simulink model "X_MEGA2560_ADVOneWire_task"  (Simulink 7.0)
libraries: logiclib x81, mathlib x64, analoglib x12, genlib x4, arclib x2, speclib x1
settings Model: Creator=Jarda  LastModifiedBy=Jarda  ExtModeTrigMode=oneshot  ExtModeArmWhenConnect=off

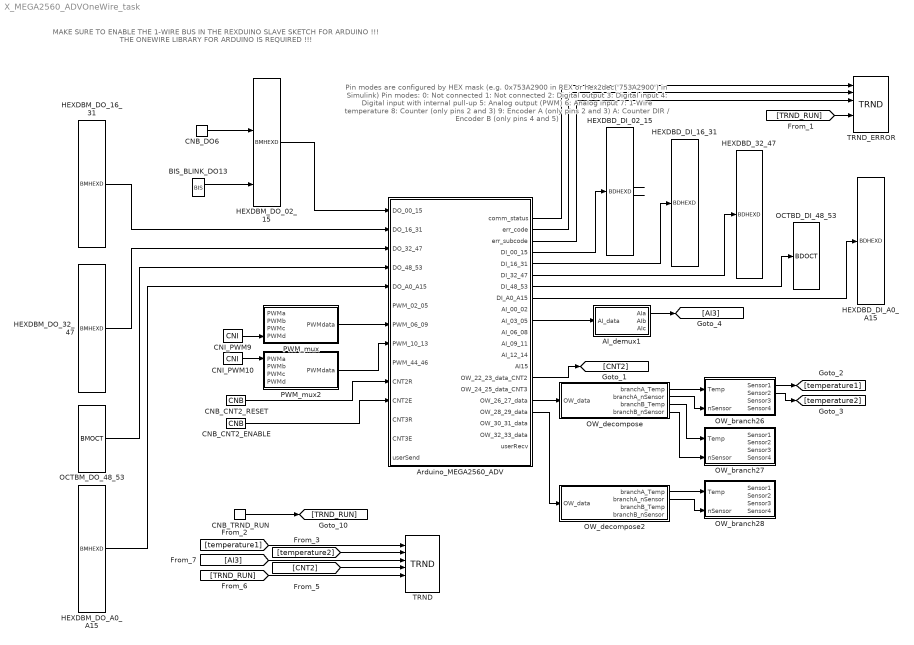
== system X_MEGA2560_ADVOneWire_task ==
  note: Pin modes are configured by HEX mask
      |    (e.g. 0x753A2900 in REX or hex2dec('753A2900') in Simulink)
      |
      | Pin modes:
      | 0: Not connected
      | 1: Not connected
      | 2: Digital output
      | 3: Digital input
      | 4: Digital input with internal pull-up
      | 5: Analog output (PWM)
      | 6: Analog input
      | 7: 1-Wire temperature
      | 8: Counter (only pins 2 and 3)
      | 9: Encoder A (only pins 2 and 3)
      | A: Counter DIR / Encoder B (only pins 4 and 5)
  note: MAKE SURE TO ENABLE THE 1-WIRE BUS IN
      | THE REXDUINO SLAVE SKETCH FOR ARDUINO !!!
      |
      | THE ONEWIRE LIBRARY FOR ARDUINO IS REQUIRED !!!
  AI_demux1 : Subsystem
      mask Type: REX sequence
  Arduino_MEGA2560_ADV : Subsystem  mask(REX sequence){comPort=/dev/ttyACM0, pinmodes_00_07=0x320A0800, pinmodes_08_15=0x00200554, pinmodes_16_23=0, pinmodes_24_31=0x00077700, pinmodes_32_39=0, pinmodes_40_47=0, pinmodes_48_53=0, pinmodes_A0_A7=0x00006000, pinmodes_A8_A15=0}
      mask prompts: comPort "Serial device, e.g. COM7, /dev/ttyACM0, /dev/ttyUSB0 etc."; pinmodes_00_07 "Pin modes 0 to 7 (0 and 1 ignored)"; pinmodes_08_15 "Pin modes 8 to 15"; pinmodes_16_23 "Pin modes 16 to 23"; pinmodes_24_31 "Pin modes 24 to 31"; pinmodes_32_39 "Pin modes 32 to 39"; pinmodes_40_47 "Pin modes 40 to 47"; pinmodes_48_53 "Pin modes 48 to 53"; pinmodes_A0_A7 "Pin modes A0 to A7"; pinmodes_A8_A15 "Pin modes A8 to A15"
      mask CallbackString:
      | REXduino_mask_comPort = get_param(gcb,'comPort');
      | REXduino_mask_comPort = sscanf(fliplr(REXduino_mask_comPort),'%u',1);
      | if ( ~isempty(REXduino_mask_comPort) & (REXduino_mask_comPort<100) )
      | set_param([gcb '/CNI_comPort'],'icn',fliplr(num2str(REXduino_mask_comPort)))
      | else
      | set_param([gcb '/CNI_comPort'],'icn','15')
      | end
      | clear REXduino_mask_comPort|||||||||
  BIS_BLINK_DO13 : genlib/BIS  Y0=off  t1=2  t2=4  t3=0  t4=4  t5=5  t6=6  t7=7  t8=8  RPT=on
  CNB_CNT2_ENABLE : mathlib/CNB  YCN=on
  CNB_CNT2_RESET : mathlib/CNB  YCN=off
  CNB_DO6 : mathlib/CNB  YCN=on
  CNB_TRND_RUN : mathlib/CNB  YCN=on
  CNI_PWM10 : mathlib/CNI  icn=128
  CNI_PWM9 : mathlib/CNI  icn=128
  HEXDBD_32_47 : logiclib/BDHEXD  shift=0
  HEXDBD_DI_02_15 : logiclib/BDHEXD  shift=0
  HEXDBD_DI_16_31 : logiclib/BDHEXD  shift=0
  HEXDBD_DI_A0_A15 : logiclib/BDHEXD  shift=0
  HEXDBM_DO_02_15 : logiclib/BMHEXD  shift=0
  HEXDBM_DO_16_31 : logiclib/BMHEXD  shift=0
  HEXDBM_DO_32_47 : logiclib/BMHEXD  shift=0
  HEXDBM_DO_A0_A15 : logiclib/BMHEXD  shift=0
  OCTBD_DI_48_53 : logiclib/BDOCT  shift=0
  OCTBM_DO_48_53 : logiclib/BMOCT  shift=0
  OW_branch26 : Subsystem
      mask Type: REX sequence
  OW_branch27 : Subsystem
      mask Type: REX sequence
  OW_branch28 : Subsystem
      mask Type: REX sequence
  OW_decompose : Subsystem
      mask Type: REX sequence
  OW_decompose2 : Subsystem
      mask Type: REX sequence
  PWM_mux : Subsystem
      mask Type: REX sequence
  PWM_mux2 : Subsystem
      mask Type: REX sequence
  TRND : arclib/TRND  n=4  l=14400  btype=8: Double  ptype1=1: Store  ptype2=1: Store  ptype3=1: Store  ptype4=1: Store  pfac=1  afac=0  arc=0  id=1  Title=Data trend
  TRND_ERROR : arclib/TRND  n=4  l=1000  btype=8: Double  ptype1=1: Store  ptype2=1: Store  ptype3=1: Store  ptype4=1: Store  pfac=1  afac=0  arc=0  id=1  Title=ERROR trend
  wires:
  AI_demux1/1(AIa) -> [AI3]
  Arduino_MEGA2560_ADV/1(comm_status) -> TRND_ERROR/1
  Arduino_MEGA2560_ADV/2(err_code) -> TRND_ERROR/2
  Arduino_MEGA2560_ADV/3(err_subcode) -> TRND_ERROR/3
  Arduino_MEGA2560_ADV/4(DI_00_15) -> HEXDBD_DI_02_15/1
  Arduino_MEGA2560_ADV/5(DI_16_31) -> HEXDBD_DI_16_31/1
  Arduino_MEGA2560_ADV/6(DI_32_47) -> HEXDBD_32_47/1
  Arduino_MEGA2560_ADV/7(DI_48_53) -> OCTBD_DI_48_53/1
  Arduino_MEGA2560_ADV/8(DI_A0_A15) -> HEXDBD_DI_A0_A15/1
  Arduino_MEGA2560_ADV/10(AI_03_05) -> AI_demux1/1(AI_data)
  Arduino_MEGA2560_ADV/15(OW_22_23_data_CNT2) -> [CNT2]
  Arduino_MEGA2560_ADV/17(OW_26_27_data) -> OW_decompose/1(OW_data)
  Arduino_MEGA2560_ADV/18(OW_28_29_data) -> OW_decompose2/1(OW_data)
  BIS_BLINK_DO13/1 -> HEXDBM_DO_02_15/14
  CNB_CNT2_ENABLE/1 -> Arduino_MEGA2560_ADV/11(CNT2E)
  CNB_CNT2_RESET/1 -> Arduino_MEGA2560_ADV/10(CNT2R)
  CNB_DO6/1 -> HEXDBM_DO_02_15/7
  CNB_TRND_RUN/1 -> [TRND_RUN]
  CNI_PWM10/1 -> PWM_mux2/1(PWMa)
  CNI_PWM9/1 -> PWM_mux/4(PWMd)
  [TRND_RUN] -> TRND_ERROR/5
  [temperature1] -> TRND/1
  [temperature2] -> TRND/2
  [CNT2] -> TRND/4
  [TRND_RUN] -> TRND/5
  [AI3] -> TRND/3
  HEXDBD_DI_02_15/8 -> ?
  HEXDBD_DI_02_15/9 -> ?
  HEXDBM_DO_02_15/1 -> Arduino_MEGA2560_ADV/1(DO_00_15)
  HEXDBM_DO_16_31/1 -> Arduino_MEGA2560_ADV/2(DO_16_31)
  HEXDBM_DO_32_47/1 -> Arduino_MEGA2560_ADV/3(DO_32_47)
  HEXDBM_DO_A0_A15/1 -> Arduino_MEGA2560_ADV/5(DO_A0_A15)
  OCTBM_DO_48_53/1 -> Arduino_MEGA2560_ADV/4(DO_48_53)
  OW_branch26/1(Sensor1) -> [temperature1]
  OW_branch26/2(Sensor2) -> [temperature2]
  OW_decompose/1(branchA_Temp) -> OW_branch26/1(Temp)
  OW_decompose/2(branchA_nSensor) -> OW_branch26/2(nSensor)
  OW_decompose/3(branchB_Temp) -> OW_branch27/1(Temp)
  OW_decompose/4(branchB_nSensor) -> OW_branch27/2(nSensor)
  OW_decompose2/1(branchA_Temp) -> OW_branch28/1(Temp)
  OW_decompose2/2(branchA_nSensor) -> OW_branch28/2(nSensor)
  PWM_mux/1(PWMdata) -> Arduino_MEGA2560_ADV/7(PWM_06_09)
  PWM_mux2/1(PWMdata) -> Arduino_MEGA2560_ADV/8(PWM_10_13)

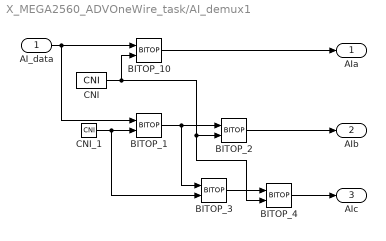
== system X_MEGA2560_ADVOneWire_task/AI_demux1 ==
  AI_data : Inport  Port=1
  BITOP_1 : logiclib/BITOP  iop=6: Shift Right
  BITOP_10 : logiclib/BITOP  iop=3: Bit AND
  BITOP_2 : logiclib/BITOP  iop=3: Bit AND
  BITOP_3 : logiclib/BITOP  iop=6: Shift Right
  BITOP_4 : logiclib/BITOP  iop=3: Bit AND
  CNI : mathlib/CNI  icn=1023
  CNI_1 : mathlib/CNI  icn=10
  AIa : Outport  Port=1
  AIb : Outport  Port=2
  AIc : Outport  Port=3
  wires:
  AI_data/1 -> BITOP_1/1, BITOP_10/1
  BITOP_1/1 -> BITOP_2/1, BITOP_3/1
  BITOP_10/1 -> AIa/1
  BITOP_2/1 -> AIb/1
  BITOP_3/1 -> BITOP_4/1
  BITOP_4/1 -> AIc/1
  CNI/1 -> BITOP_10/2, BITOP_2/2, BITOP_4/2
  CNI_1/1 -> BITOP_1/2, BITOP_3/2

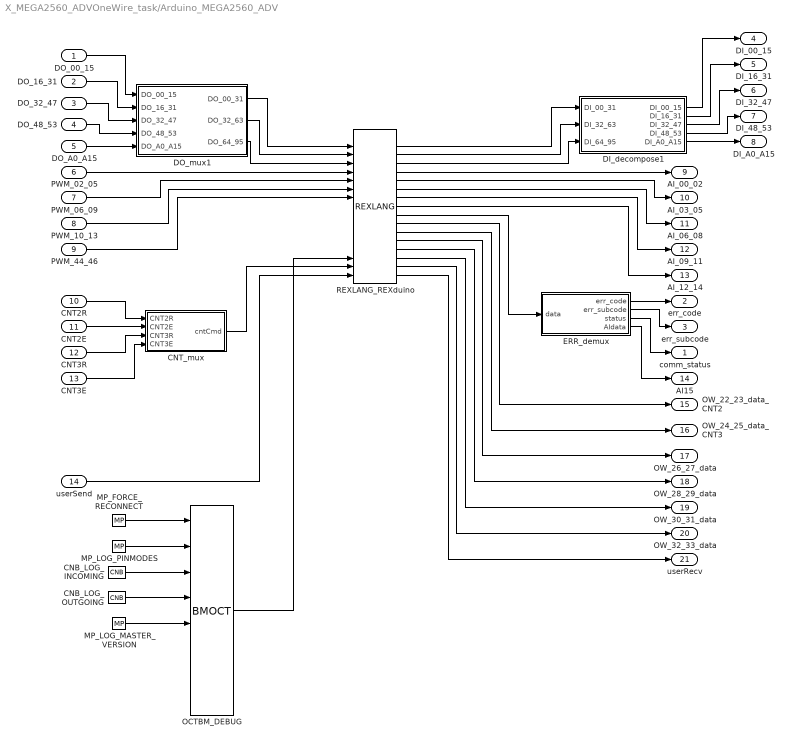
== system X_MEGA2560_ADVOneWire_task/Arduino_MEGA2560_ADV ==
  DO_00_15 : Inport  Port=1  PortWidth=-1  SampleTime=-1  DataType=auto
      settings: SignalType=auto
  DO_16_31 : Inport  Port=2  PortWidth=-1  SampleTime=-1  DataType=auto
      settings: SignalType=auto
  DO_32_47 : Inport  Port=3  PortWidth=-1  SampleTime=-1  DataType=auto
      settings: SignalType=auto
  DO_48_53 : Inport  Port=4  PortWidth=-1  SampleTime=-1  DataType=auto
      settings: SignalType=auto
  DO_A0_A15 : Inport  Port=5  PortWidth=-1  SampleTime=-1  DataType=auto
      settings: SignalType=auto
  PWM_02_05 : Inport  Port=6  PortWidth=-1  SampleTime=-1  DataType=auto
      settings: SignalType=auto
  PWM_06_09 : Inport  Port=7  PortWidth=-1  SampleTime=-1  DataType=auto
      settings: SignalType=auto
  PWM_10_13 : Inport  Port=8  PortWidth=-1  SampleTime=-1  DataType=auto
      settings: SignalType=auto
  PWM_44_46 : Inport  Port=9  PortWidth=-1  SampleTime=-1  DataType=auto
      settings: SignalType=auto
  CNT2R : Inport  Port=10  PortWidth=-1  SampleTime=-1  DataType=auto
      settings: SignalType=auto
  CNT2E : Inport  Port=11  PortWidth=-1  SampleTime=-1  DataType=auto
      settings: SignalType=auto
  CNT3R : Inport  Port=12  PortWidth=-1  SampleTime=-1  DataType=auto
      settings: SignalType=auto
  CNT3E : Inport  Port=13  PortWidth=-1  SampleTime=-1  DataType=auto
      settings: SignalType=auto
  userSend : Inport  Port=14  PortWidth=-1  SampleTime=-1  DataType=auto
      settings: SignalType=auto
  CNB_LOG_INCOMING : mathlib/CNB  SystemSampleTime=-1  YCN=off
  CNB_LOG_OUTGOING : mathlib/CNB  SystemSampleTime=-1  YCN=off
  CNT_mux : Subsystem
      mask Type: REX sequence
  DI_decompose1 : Subsystem
      mask Type: REX sequence
  DO_mux1 : Subsystem
      mask Type: REX sequence
  ERR_demux : Subsystem
      mask Type: REX sequence
  MP_FORCE_RECONNECT : genlib/MP  SystemSampleTime=-1  pwidth=10  BSTATE=off  RPTF=off
  MP_LOG_MASTER_VERSION : genlib/MP  SystemSampleTime=-1  pwidth=10  BSTATE=off  RPTF=off
  MP_LOG_PINMODES : genlib/MP  SystemSampleTime=-1  pwidth=10  BSTATE=off  RPTF=off
  OCTBM_DEBUG : logiclib/BMOCT  SystemSampleTime=-1  shift=0
  REXLANG_REXduino : speclib/REXLANG  tab_matlab=MORE  srcname=REXduino_master.stl  srctype=1: STL  stack=0  debug=1: No check  fname=comPort  p0=0  p1=pinmodes_00_07  p2=pinmodes_08_15  p3=pinmodes_16_23  p4=pinmodes_24_31  p5=pinmodes_32_39  p6=pinmodes_40_47  p7=pinmodes_48_53  p8=pinmodes_A0_A7  p9=pinmodes_A8_A15  p10=0  p11=0  p12=0  p13=0  p14=0  p15=4
  comm_status : Outport  Port=1
  err_code : Outport  Port=2
  err_subcode : Outport  Port=3
  DI_00_15 : Outport  Port=4
  DI_16_31 : Outport  Port=5
  DI_32_47 : Outport  Port=6
  DI_48_53 : Outport  Port=7
  DI_A0_A15 : Outport  Port=8
  AI_00_02 : Outport  Port=9
  AI_03_05 : Outport  Port=10
  AI_06_08 : Outport  Port=11
  AI_09_11 : Outport  Port=12
  AI_12_14 : Outport  Port=13
  AI15 : Outport  Port=14
  OW_22_23_data_CNT2 : Outport  Port=15
  OW_24_25_data_CNT3 : Outport  Port=16
  OW_26_27_data : Outport  Port=17
  OW_28_29_data : Outport  Port=18
  OW_30_31_data : Outport  Port=19
  OW_32_33_data : Outport  Port=20
  userRecv : Outport  Port=21
  wires:
  CNB_LOG_INCOMING/1 -> OCTBM_DEBUG/3
  CNB_LOG_OUTGOING/1 -> OCTBM_DEBUG/4
  CNT2E/1 -> CNT_mux/2(CNT2E)
  CNT2R/1 -> CNT_mux/1(CNT2R)
  CNT3E/1 -> CNT_mux/4(CNT3E)
  CNT3R/1 -> CNT_mux/3(CNT3R)
  CNT_mux/1(cntCmd) -> REXLANG_REXduino/16
  DI_decompose1/1(DI_00_15) -> DI_00_15/1
  DI_decompose1/2(DI_16_31) -> DI_16_31/1
  DI_decompose1/3(DI_32_47) -> DI_32_47/1
  DI_decompose1/4(DI_48_53) -> DI_48_53/1
  DI_decompose1/5(DI_A0_A15) -> DI_A0_A15/1
  DO_00_15/1 -> DO_mux1/1(DO_00_15)
  DO_16_31/1 -> DO_mux1/2(DO_16_31)
  DO_32_47/1 -> DO_mux1/3(DO_32_47)
  DO_48_53/1 -> DO_mux1/4(DO_48_53)
  DO_A0_A15/1 -> DO_mux1/5(DO_A0_A15)
  DO_mux1/1(DO_00_31) -> REXLANG_REXduino/2
  DO_mux1/2(DO_32_63) -> REXLANG_REXduino/3
  DO_mux1/3(DO_64_95) -> REXLANG_REXduino/4
  ERR_demux/1(err_code) -> err_code/1
  ERR_demux/2(err_subcode) -> err_subcode/1
  ERR_demux/3(status) -> comm_status/1
  ERR_demux/4(AIdata) -> AI15/1
  MP_FORCE_RECONNECT/1 -> OCTBM_DEBUG/1
  MP_LOG_MASTER_VERSION/1 -> OCTBM_DEBUG/5
  MP_LOG_PINMODES/1 -> OCTBM_DEBUG/2
  OCTBM_DEBUG/1 -> REXLANG_REXduino/15
  PWM_02_05/1 -> REXLANG_REXduino/5
  PWM_06_09/1 -> REXLANG_REXduino/6
  PWM_10_13/1 -> REXLANG_REXduino/7
  PWM_44_46/1 -> REXLANG_REXduino/8
  REXLANG_REXduino/2 -> DI_decompose1/1(DI_00_31)
  REXLANG_REXduino/3 -> DI_decompose1/2(DI_32_63)
  REXLANG_REXduino/4 -> DI_decompose1/3(DI_64_95)
  REXLANG_REXduino/5 -> AI_00_02/1
  REXLANG_REXduino/6 -> AI_03_05/1
  REXLANG_REXduino/7 -> AI_06_08/1
  REXLANG_REXduino/8 -> AI_09_11/1
  REXLANG_REXduino/9 -> AI_12_14/1
  REXLANG_REXduino/10 -> ERR_demux/1(data)
  REXLANG_REXduino/11 -> OW_22_23_data_CNT2/1
  REXLANG_REXduino/12 -> OW_24_25_data_CNT3/1
  REXLANG_REXduino/13 -> OW_26_27_data/1
  REXLANG_REXduino/14 -> OW_28_29_data/1
  REXLANG_REXduino/15 -> OW_30_31_data/1
  REXLANG_REXduino/16 -> OW_32_33_data/1
  REXLANG_REXduino/17 -> userRecv/1
  userSend/1 -> REXLANG_REXduino/17

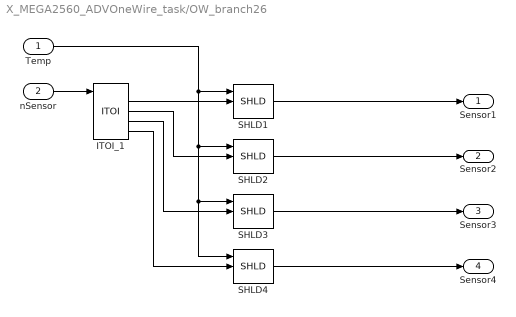
== system X_MEGA2560_ADVOneWire_task/OW_branch26 ==
  Temp : Inport  Port=1  PortWidth=-1  SampleTime=-1  DataType=auto
      settings: SignalType=auto
  nSensor : Inport  Port=2  PortWidth=-1  SampleTime=-1  DataType=auto
      settings: SignalType=auto
  ITOI_1 : logiclib/ITOI  BINF=off  fktab=[0 1 2 4 8 0 0 0 0 0 0 0 0 0 0 0]
  SHLD{1..4} (4 alike) : analoglib/SHLD  y0=0  mode=1: Triggered sampling
  Sensor1 : Outport  Port=1
  Sensor2 : Outport  Port=2
  Sensor3 : Outport  Port=3
  Sensor4 : Outport  Port=4
  wires:
  ITOI_1/2 -> SHLD1/2
  ITOI_1/3 -> SHLD2/2
  ITOI_1/4 -> SHLD3/2
  ITOI_1/5 -> SHLD4/2
  SHLD1/1 -> Sensor1/1
  SHLD2/1 -> Sensor2/1
  SHLD3/1 -> Sensor3/1
  SHLD4/1 -> Sensor4/1
  Temp/1 -> SHLD3/1, SHLD4/1, SHLD2/1, SHLD1/1
  nSensor/1 -> ITOI_1/1

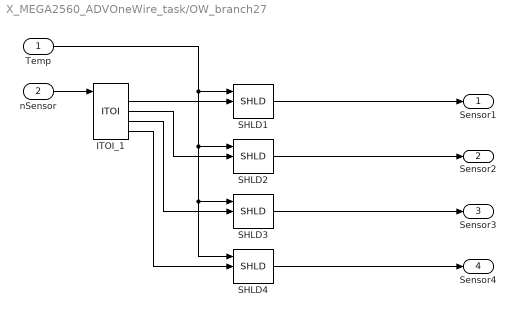
== system X_MEGA2560_ADVOneWire_task/OW_branch27 ==
  Temp : Inport  Port=1  PortWidth=-1  SampleTime=-1  DataType=auto
      settings: SignalType=auto
  nSensor : Inport  Port=2  PortWidth=-1  SampleTime=-1  DataType=auto
      settings: SignalType=auto
  ITOI_1 : logiclib/ITOI  BINF=off  fktab=[0 1 2 4 8 0 0 0 0 0 0 0 0 0 0 0]
  SHLD{1..4} (4 alike) : analoglib/SHLD  y0=0  mode=1: Triggered sampling
  Sensor1 : Outport  Port=1
  Sensor2 : Outport  Port=2
  Sensor3 : Outport  Port=3
  Sensor4 : Outport  Port=4
  wires:
  ITOI_1/2 -> SHLD1/2
  ITOI_1/3 -> SHLD2/2
  ITOI_1/4 -> SHLD3/2
  ITOI_1/5 -> SHLD4/2
  SHLD1/1 -> Sensor1/1
  SHLD2/1 -> Sensor2/1
  SHLD3/1 -> Sensor3/1
  SHLD4/1 -> Sensor4/1
  Temp/1 -> SHLD3/1, SHLD4/1, SHLD2/1, SHLD1/1
  nSensor/1 -> ITOI_1/1

== system X_MEGA2560_ADVOneWire_task/OW_branch28 ==
  Temp : Inport  Port=1  PortWidth=-1  SampleTime=-1  DataType=auto
      settings: SignalType=auto
  nSensor : Inport  Port=2  PortWidth=-1  SampleTime=-1  DataType=auto
      settings: SignalType=auto
  ITOI_1 : logiclib/ITOI  BINF=off  fktab=[0 1 2 4 8 0 0 0 0 0 0 0 0 0 0 0]
  SHLD{1..4} (4 alike) : analoglib/SHLD  y0=0  mode=1: Triggered sampling
  Sensor1 : Outport  Port=1
  Sensor2 : Outport  Port=2
  Sensor3 : Outport  Port=3
  Sensor4 : Outport  Port=4
  wires:
  ITOI_1/2 -> SHLD1/2
  ITOI_1/3 -> SHLD2/2
  ITOI_1/4 -> SHLD3/2
  ITOI_1/5 -> SHLD4/2
  SHLD1/1 -> Sensor1/1
  SHLD2/1 -> Sensor2/1
  SHLD3/1 -> Sensor3/1
  SHLD4/1 -> Sensor4/1
  Temp/1 -> SHLD3/1, SHLD4/1, SHLD2/1, SHLD1/1
  nSensor/1 -> ITOI_1/1

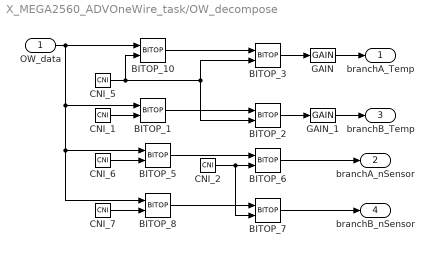
== system X_MEGA2560_ADVOneWire_task/OW_decompose ==
  OW_data : Inport  Port=1
  BITOP_1 : logiclib/BITOP  iop=5: Shift Left
  BITOP_10 : logiclib/BITOP  iop=5: Shift Left
  BITOP_{2..3,5,8} (4 alike) : logiclib/BITOP  iop=6: Shift Right
  BITOP_6 : logiclib/BITOP  iop=3: Bit AND
  BITOP_7 : logiclib/BITOP  iop=3: Bit AND
  CNI_1 : mathlib/CNI  icn=4
  CNI_2 : mathlib/CNI  icn=15
  CNI_5 : mathlib/CNI  icn=20
  CNI_6 : mathlib/CNI  icn=12
  CNI_7 : mathlib/CNI  icn=28
  GAIN : mathlib/GAIN  k=0.0625
  GAIN_1 : mathlib/GAIN  k=0.0625
  branchA_Temp : Outport  Port=1
  branchA_nSensor : Outport  Port=2
  branchB_Temp : Outport  Port=3
  branchB_nSensor : Outport  Port=4
  wires:
  BITOP_1/1 -> BITOP_2/1
  BITOP_10/1 -> BITOP_3/1
  BITOP_2/1 -> GAIN_1/1
  BITOP_3/1 -> GAIN/1
  BITOP_5/1 -> BITOP_6/1
  BITOP_6/1 -> branchA_nSensor/1
  BITOP_7/1 -> branchB_nSensor/1
  BITOP_8/1 -> BITOP_7/1
  CNI_1/1 -> BITOP_1/2
  CNI_2/1 -> BITOP_6/2, BITOP_7/2
  CNI_5/1 -> BITOP_10/2, BITOP_2/2, BITOP_3/2
  CNI_6/1 -> BITOP_5/2
  CNI_7/1 -> BITOP_8/2
  GAIN/1 -> branchA_Temp/1
  GAIN_1/1 -> branchB_Temp/1
  OW_data/1 -> BITOP_10/1, BITOP_1/1, BITOP_5/1, BITOP_8/1

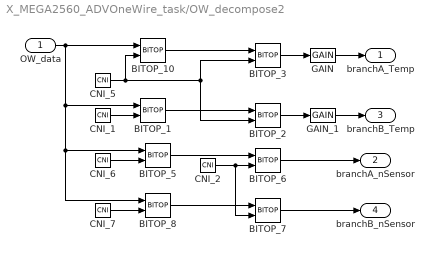
== system X_MEGA2560_ADVOneWire_task/OW_decompose2 ==
  OW_data : Inport  Port=1
  BITOP_1 : logiclib/BITOP  iop=5: Shift Left
  BITOP_10 : logiclib/BITOP  iop=5: Shift Left
  BITOP_{2..3,5,8} (4 alike) : logiclib/BITOP  iop=6: Shift Right
  BITOP_6 : logiclib/BITOP  iop=3: Bit AND
  BITOP_7 : logiclib/BITOP  iop=3: Bit AND
  CNI_1 : mathlib/CNI  icn=4
  CNI_2 : mathlib/CNI  icn=15
  CNI_5 : mathlib/CNI  icn=20
  CNI_6 : mathlib/CNI  icn=12
  CNI_7 : mathlib/CNI  icn=28
  GAIN : mathlib/GAIN  k=0.0625
  GAIN_1 : mathlib/GAIN  k=0.0625
  branchA_Temp : Outport  Port=1
  branchA_nSensor : Outport  Port=2
  branchB_Temp : Outport  Port=3
  branchB_nSensor : Outport  Port=4
  wires:
  BITOP_1/1 -> BITOP_2/1
  BITOP_10/1 -> BITOP_3/1
  BITOP_2/1 -> GAIN_1/1
  BITOP_3/1 -> GAIN/1
  BITOP_5/1 -> BITOP_6/1
  BITOP_6/1 -> branchA_nSensor/1
  BITOP_7/1 -> branchB_nSensor/1
  BITOP_8/1 -> BITOP_7/1
  CNI_1/1 -> BITOP_1/2
  CNI_2/1 -> BITOP_6/2, BITOP_7/2
  CNI_5/1 -> BITOP_10/2, BITOP_2/2, BITOP_3/2
  CNI_6/1 -> BITOP_5/2
  CNI_7/1 -> BITOP_8/2
  GAIN/1 -> branchA_Temp/1
  GAIN_1/1 -> branchB_Temp/1
  OW_data/1 -> BITOP_10/1, BITOP_1/1, BITOP_5/1, BITOP_8/1

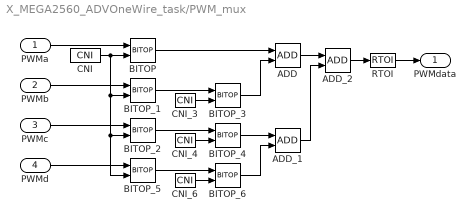
== system X_MEGA2560_ADVOneWire_task/PWM_mux ==
  PWMa : Inport  Port=1
  PWMb : Inport  Port=2
  PWMc : Inport  Port=3
  PWMd : Inport  Port=4
  ADD : mathlib/ADD
  ADD_1 : mathlib/ADD
  ADD_2 : mathlib/ADD
  BITOP : logiclib/BITOP  iop=3: Bit AND
  BITOP_1 : logiclib/BITOP  iop=3: Bit AND
  BITOP_2 : logiclib/BITOP  iop=3: Bit AND
  BITOP_3 : logiclib/BITOP  iop=5: Shift Left
  BITOP_4 : logiclib/BITOP  iop=5: Shift Left
  BITOP_5 : logiclib/BITOP  iop=3: Bit AND
  BITOP_6 : logiclib/BITOP  iop=5: Shift Left
  CNI : mathlib/CNI  icn=255
  CNI_3 : mathlib/CNI  icn=8
  CNI_4 : mathlib/CNI  icn=16
  CNI_6 : mathlib/CNI  icn=24
  RTOI : mathlib/RTOI
  PWMdata : Outport  Port=1
  wires:
  ADD/1 -> ADD_2/1
  ADD_1/1 -> ADD_2/2
  ADD_2/1 -> RTOI/1
  BITOP/1 -> ADD/1
  BITOP_1/1 -> BITOP_3/1
  BITOP_2/1 -> BITOP_4/1
  BITOP_3/1 -> ADD/2
  BITOP_4/1 -> ADD_1/1
  BITOP_5/1 -> BITOP_6/1
  BITOP_6/1 -> ADD_1/2
  CNI/1 -> BITOP/2, BITOP_1/2, BITOP_2/2, BITOP_5/2
  CNI_3/1 -> BITOP_3/2
  CNI_4/1 -> BITOP_4/2
  CNI_6/1 -> BITOP_6/2
  PWMa/1 -> BITOP/1
  PWMb/1 -> BITOP_1/1
  PWMc/1 -> BITOP_2/1
  PWMd/1 -> BITOP_5/1
  RTOI/1 -> PWMdata/1

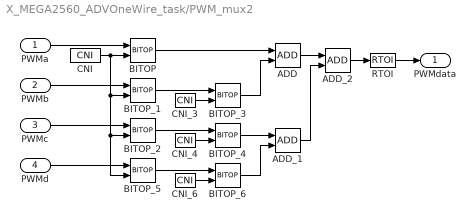
== system X_MEGA2560_ADVOneWire_task/PWM_mux2 ==
  PWMa : Inport  Port=1
  PWMb : Inport  Port=2
  PWMc : Inport  Port=3
  PWMd : Inport  Port=4
  ADD : mathlib/ADD
  ADD_1 : mathlib/ADD
  ADD_2 : mathlib/ADD
  BITOP : logiclib/BITOP  iop=3: Bit AND
  BITOP_1 : logiclib/BITOP  iop=3: Bit AND
  BITOP_2 : logiclib/BITOP  iop=3: Bit AND
  BITOP_3 : logiclib/BITOP  iop=5: Shift Left
  BITOP_4 : logiclib/BITOP  iop=5: Shift Left
  BITOP_5 : logiclib/BITOP  iop=3: Bit AND
  BITOP_6 : logiclib/BITOP  iop=5: Shift Left
  CNI : mathlib/CNI  icn=255
  CNI_3 : mathlib/CNI  icn=8
  CNI_4 : mathlib/CNI  icn=16
  CNI_6 : mathlib/CNI  icn=24
  RTOI : mathlib/RTOI
  PWMdata : Outport  Port=1
  wires:
  ADD/1 -> ADD_2/1
  ADD_1/1 -> ADD_2/2
  ADD_2/1 -> RTOI/1
  BITOP/1 -> ADD/1
  BITOP_1/1 -> BITOP_3/1
  BITOP_2/1 -> BITOP_4/1
  BITOP_3/1 -> ADD/2
  BITOP_4/1 -> ADD_1/1
  BITOP_5/1 -> BITOP_6/1
  BITOP_6/1 -> ADD_1/2
  CNI/1 -> BITOP/2, BITOP_1/2, BITOP_2/2, BITOP_5/2
  CNI_3/1 -> BITOP_3/2
  CNI_4/1 -> BITOP_4/2
  CNI_6/1 -> BITOP_6/2
  PWMa/1 -> BITOP/1
  PWMb/1 -> BITOP_1/1
  PWMc/1 -> BITOP_2/1
  PWMd/1 -> BITOP_5/1
  RTOI/1 -> PWMdata/1

== system X_MEGA2560_ADVOneWire_task/Arduino_MEGA2560_ADV/CNT_mux ==
  CNT2R : Inport  Port=1  PortWidth=-1  SampleTime=-1  DataType=auto
      settings: SignalType=auto
  CNT2E : Inport  Port=2  PortWidth=-1  SampleTime=-1  DataType=auto
      settings: SignalType=auto
  CNT3R : Inport  Port=3  PortWidth=-1  SampleTime=-1  DataType=auto
      settings: SignalType=auto
  CNT3E : Inport  Port=4  PortWidth=-1  SampleTime=-1  DataType=auto
      settings: SignalType=auto
  OCTBM : logiclib/BMOCT  shift=0
  cntCmd : Outport  Port=1
  wires:
  CNT2E/1 -> OCTBM/2
  CNT2R/1 -> OCTBM/1
  CNT3E/1 -> OCTBM/4
  CNT3R/1 -> OCTBM/3
  OCTBM/1 -> cntCmd/1

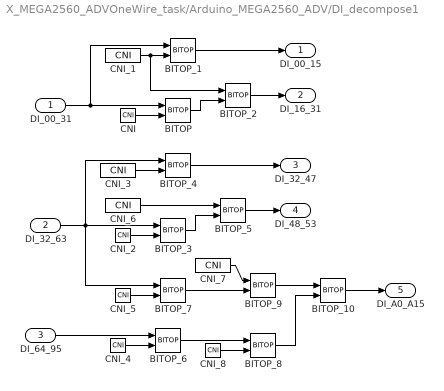
== system X_MEGA2560_ADVOneWire_task/Arduino_MEGA2560_ADV/DI_decompose1 ==
  DI_00_31 : Inport  Port=1  PortWidth=-1  SampleTime=-1  DataType=auto
      settings: SignalType=auto
  DI_32_63 : Inport  Port=2  PortWidth=-1  SampleTime=-1  DataType=auto
      settings: SignalType=auto
  DI_64_95 : Inport  Port=3  PortWidth=-1  SampleTime=-1  DataType=auto
      settings: SignalType=auto
  BITOP : logiclib/BITOP  iop=6: Shift Right
  BITOP_{1..2,4..6,9} (6 alike) : logiclib/BITOP  iop=3: Bit AND
  BITOP_10 : logiclib/BITOP  iop=2: Bit OR
  BITOP_3 : logiclib/BITOP  iop=6: Shift Right
  BITOP_7 : logiclib/BITOP  iop=6: Shift Right
  BITOP_8 : logiclib/BITOP  iop=5: Shift Left
  CNI : mathlib/CNI  icn=16
  CNI_1 : mathlib/CNI  icn=65535
  CNI_2 : mathlib/CNI  icn=16
  CNI_3 : mathlib/CNI  icn=65535
  CNI_4 : mathlib/CNI  icn=63
  CNI_5 : mathlib/CNI  icn=22
  CNI_6 : mathlib/CNI  icn=63
  CNI_7 : mathlib/CNI  icn=1023
  CNI_8 : mathlib/CNI  icn=10
  DI_00_15 : Outport  Port=1
  DI_16_31 : Outport  Port=2
  DI_32_47 : Outport  Port=3
  DI_48_53 : Outport  Port=4
  DI_A0_A15 : Outport  Port=5
  wires:
  BITOP/1 -> BITOP_2/2
  BITOP_1/1 -> DI_00_15/1
  BITOP_10/1 -> DI_A0_A15/1
  BITOP_2/1 -> DI_16_31/1
  BITOP_3/1 -> BITOP_5/2
  BITOP_4/1 -> DI_32_47/1
  BITOP_5/1 -> DI_48_53/1
  BITOP_6/1 -> BITOP_8/1
  BITOP_7/1 -> BITOP_9/2
  BITOP_8/1 -> BITOP_10/2
  BITOP_9/1 -> BITOP_10/1
  CNI/1 -> BITOP/2
  CNI_1/1 -> BITOP_1/2, BITOP_2/1
  CNI_2/1 -> BITOP_3/2
  CNI_3/1 -> BITOP_4/2
  CNI_4/1 -> BITOP_6/2
  CNI_5/1 -> BITOP_7/2
  CNI_6/1 -> BITOP_5/1
  CNI_7/1 -> BITOP_9/1
  CNI_8/1 -> BITOP_8/2
  DI_00_31/1 -> BITOP/1, BITOP_1/1
  DI_32_63/1 -> BITOP_3/1, BITOP_4/1, BITOP_7/1
  DI_64_95/1 -> BITOP_6/1

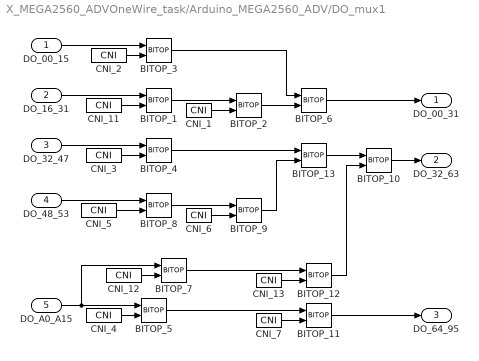
== system X_MEGA2560_ADVOneWire_task/Arduino_MEGA2560_ADV/DO_mux1 ==
  DO_00_15 : Inport  Port=1  PortWidth=-1  SampleTime=-1  DataType=auto
      settings: SignalType=auto
  DO_16_31 : Inport  Port=2  PortWidth=-1  SampleTime=-1  DataType=auto
      settings: SignalType=auto
  DO_32_47 : Inport  Port=3  PortWidth=-1  SampleTime=-1  DataType=auto
      settings: SignalType=auto
  DO_48_53 : Inport  Port=4  PortWidth=-1  SampleTime=-1  DataType=auto
      settings: SignalType=auto
  DO_A0_A15 : Inport  Port=5  PortWidth=-1  SampleTime=-1  DataType=auto
      settings: SignalType=auto
  BITOP_{1,3..5,7..8} (6 alike) : logiclib/BITOP  iop=3: Bit AND
  BITOP_10 : logiclib/BITOP  iop=2: Bit OR
  BITOP_11 : logiclib/BITOP  iop=6: Shift Right
  BITOP_12 : logiclib/BITOP  iop=5: Shift Left
  BITOP_13 : logiclib/BITOP  iop=2: Bit OR
  BITOP_2 : logiclib/BITOP  iop=5: Shift Left
  BITOP_6 : logiclib/BITOP  iop=2: Bit OR
  BITOP_9 : logiclib/BITOP  iop=5: Shift Left
  CNI_1 : mathlib/CNI  icn=16
  CNI_11 : mathlib/CNI  icn=65535
  CNI_12 : mathlib/CNI  icn=1023
  CNI_13 : mathlib/CNI  icn=22
  CNI_2 : mathlib/CNI  icn=65535
  CNI_3 : mathlib/CNI  icn=65535
  CNI_4 : mathlib/CNI  icn=64512
  CNI_5 : mathlib/CNI  icn=63
  CNI_6 : mathlib/CNI  icn=16
  CNI_7 : mathlib/CNI  icn=10
  DO_00_31 : Outport  Port=1
  DO_32_63 : Outport  Port=2
  DO_64_95 : Outport  Port=3
  wires:
  BITOP_1/1 -> BITOP_2/1
  BITOP_10/1 -> DO_32_63/1
  BITOP_11/1 -> DO_64_95/1
  BITOP_12/1 -> BITOP_10/2
  BITOP_13/1 -> BITOP_10/1
  BITOP_2/1 -> BITOP_6/2
  BITOP_3/1 -> BITOP_6/1
  BITOP_4/1 -> BITOP_13/1
  BITOP_5/1 -> BITOP_11/1
  BITOP_6/1 -> DO_00_31/1
  BITOP_7/1 -> BITOP_12/1
  BITOP_8/1 -> BITOP_9/1
  BITOP_9/1 -> BITOP_13/2
  CNI_1/1 -> BITOP_2/2
  CNI_11/1 -> BITOP_1/2
  CNI_12/1 -> BITOP_7/2
  CNI_13/1 -> BITOP_12/2
  CNI_2/1 -> BITOP_3/2
  CNI_3/1 -> BITOP_4/2
  CNI_4/1 -> BITOP_5/2
  CNI_5/1 -> BITOP_8/2
  CNI_6/1 -> BITOP_9/2
  CNI_7/1 -> BITOP_11/2
  DO_00_15/1 -> BITOP_3/1
  DO_16_31/1 -> BITOP_1/1
  DO_32_47/1 -> BITOP_4/1
  DO_48_53/1 -> BITOP_8/1
  DO_A0_A15/1 -> BITOP_5/1, BITOP_7/1

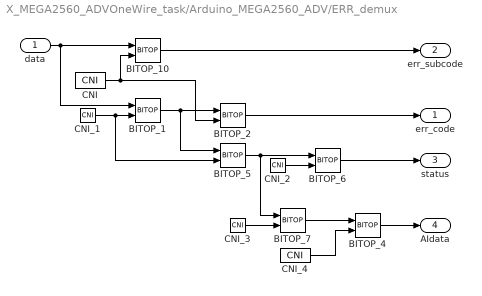
== system X_MEGA2560_ADVOneWire_task/Arduino_MEGA2560_ADV/ERR_demux ==
  data : Inport  Port=1  PortWidth=-1  SampleTime=-1  DataType=auto
      settings: SignalType=auto
  BITOP_1 : logiclib/BITOP  iop=6: Shift Right
  BITOP_{2,4,6,10} (4 alike) : logiclib/BITOP  iop=3: Bit AND
  BITOP_5 : logiclib/BITOP  iop=6: Shift Right
  BITOP_7 : logiclib/BITOP  iop=6: Shift Right
  CNI : mathlib/CNI  icn=255
  CNI_1 : mathlib/CNI  icn=8
  CNI_2 : mathlib/CNI  icn=63
  CNI_3 : mathlib/CNI  icn=6
  CNI_4 : mathlib/CNI  icn=1023
  err_code : Outport  Port=1
  err_subcode : Outport  Port=2
  status : Outport  Port=3
  AIdata : Outport  Port=4
  wires:
  BITOP_1/1 -> BITOP_2/1, BITOP_5/1
  BITOP_10/1 -> err_subcode/1
  BITOP_2/1 -> err_code/1
  BITOP_4/1 -> AIdata/1
  BITOP_5/1 -> BITOP_6/1, BITOP_7/1
  BITOP_6/1 -> status/1
  BITOP_7/1 -> BITOP_4/1
  CNI/1 -> BITOP_10/2, BITOP_2/2
  CNI_1/1 -> BITOP_1/2, BITOP_5/2
  CNI_2/1 -> BITOP_6/2
  CNI_3/1 -> BITOP_7/2
  CNI_4/1 -> BITOP_4/2
  data/1 -> BITOP_1/1, BITOP_10/1
